simulink model "Cinematica_MGI"  (Simulink 7.7)
settings: Solver=ode45  StartTime=0.0  StopTime=inf  RelTol=1e-3
libraries: simulink x4
settings Model: Creator=JohnConstantine  LastModifiedBy=JohnConstantine

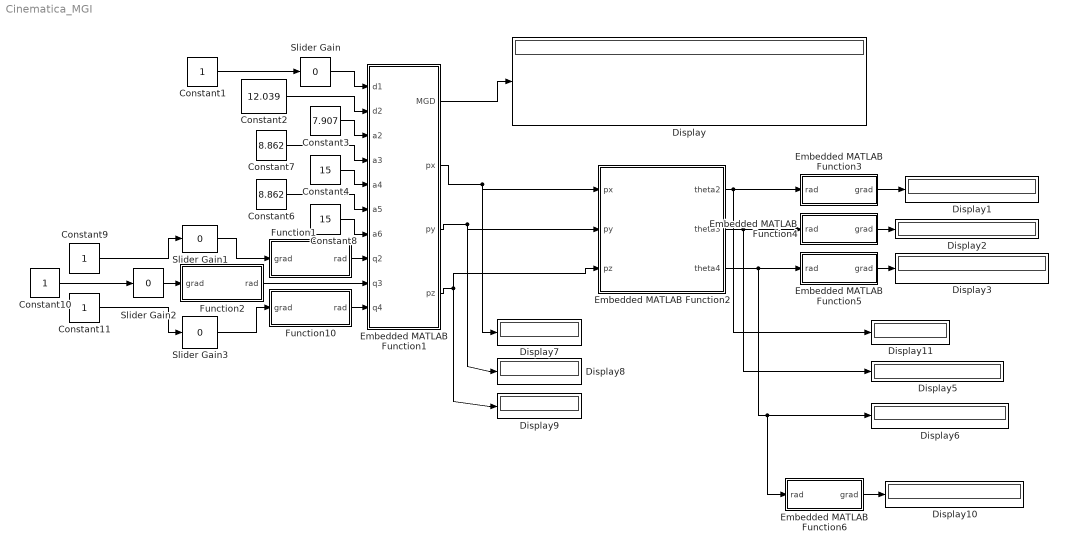
== system Cinematica_MGI ==
  Constant{1,9..11} (4 alike) : Constant
  Constant2 : Constant  Value=12.039
  Constant3 : Constant  Value=7.907
  Constant4 : Constant  Value=15
  Constant6 : Constant  Value=8.862
  Constant7 : Constant  Value=8.862
  Constant8 : Constant  Value=15
  Display{,1..3,5..11} (11 alike) : Display
  Embedded MATLAB Function1 : Stateflow chart  TreatAsAtomicUnit=on
  Embedded MATLAB Function2 : Stateflow chart  TreatAsAtomicUnit=on
  Embedded MATLAB Function3 : Stateflow chart  TreatAsAtomicUnit=on
  Embedded MATLAB Function4 : Stateflow chart  TreatAsAtomicUnit=on
  Embedded MATLAB Function5 : Stateflow chart  TreatAsAtomicUnit=on
  Embedded MATLAB Function6 : Stateflow chart  TreatAsAtomicUnit=on
  Function1 : Stateflow chart  TreatAsAtomicUnit=on
  Function10 : Stateflow chart  TreatAsAtomicUnit=on
  Function2 : Stateflow chart  TreatAsAtomicUnit=on
  Slider Gain : simulink/Math Operations/Slider Gain  SystemSampleTime=-1  low=0  gain=0  high=25
  Slider Gain1 : simulink/Math Operations/Slider Gain  SystemSampleTime=-1  low=0  gain=0  high=15
  Slider Gain2 : simulink/Math Operations/Slider Gain  SystemSampleTime=-1  low=0  gain=0  high=90
  Slider Gain3 : simulink/Math Operations/Slider Gain  SystemSampleTime=-1  low=0  gain=0  high=110
  wires:
  Embedded MATLAB Function1/2(px) -> Display7/1, Embedded MATLAB Function2/1(px)
  Embedded MATLAB Function1/1(MGD) -> Display/1
  Slider Gain/1 -> Embedded MATLAB Function1/1(d1)
  Constant4/1 -> Embedded MATLAB Function1/5(a4)
  Constant3/1 -> Embedded MATLAB Function1/3(a2)
  Constant8/1 -> Embedded MATLAB Function1/7(a6)
  Constant6/1 -> Embedded MATLAB Function1/6(a5)
  Constant7/1 -> Embedded MATLAB Function1/4(a3)
  Constant2/1 -> Embedded MATLAB Function1/2(d2)
  Embedded MATLAB Function2/1(theta2) -> Embedded MATLAB Function3/1(rad), Display11/1
  Embedded MATLAB Function2/2(theta3) -> Embedded MATLAB Function4/1(rad), Display5/1
  Embedded MATLAB Function2/3(theta4) -> Embedded MATLAB Function5/1(rad), Display6/1, Embedded MATLAB Function6/1(rad)
  Embedded MATLAB Function1/3(py) -> Display8/1, Embedded MATLAB Function2/2(py)
  Embedded MATLAB Function1/4(pz) -> Display9/1, Embedded MATLAB Function2/3(pz)
  Constant1/1 -> Slider Gain/1
  Constant9/1 -> Slider Gain1/1
  Constant10/1 -> Slider Gain2/1
  Constant11/1 -> Slider Gain3/1
  Embedded MATLAB Function3/1(grad) -> Display1/1
  Embedded MATLAB Function4/1(grad) -> Display2/1
  Embedded MATLAB Function5/1(grad) -> Display3/1
  Embedded MATLAB Function6/1(grad) -> Display10/1
  Slider Gain1/1 -> Function1/1(grad)
  Function1/1(rad) -> Embedded MATLAB Function1/8(q2)
  Function2/1(rad) -> Embedded MATLAB Function1/9(q3)
  Function10/1(rad) -> Embedded MATLAB Function1/10(q4)
  Slider Gain3/1 -> Function10/1(grad)
  Slider Gain2/1 -> Function2/1(grad)

== matlab function Embedded MATLAB Function1 ==
  data: d1 input double; MGD output double; d2 input double; a2 input double; a3 input double; a4 input double; a5 input double; a6 input double; q2 input double; q3 input double; q4 input double; px output double; py output double; pz output double
function [MGD,px,py,pz] =mgdFalange(d1,d2,a2,a3,a4,a5,a6,q2,q3,q4)

MGD= [ cos(q3)*cos(q4)*cos(pi/2 + q2) - cos(pi/2 + q2)*sin(q3)*sin(q4), - cos(q3)*cos(pi/2 + q2)*sin(q4) - cos(q4)*cos(pi/2 + q2)*sin(q3),  sin(pi/2 + q2),      a2*cos(pi/2 + q2) + cos(q3)*cos(pi/2 + q2)*(a3 + a4) + cos(q3)*cos(q4)*cos(pi/2 + q2)*(a5 + a6) - cos(pi/2 + q2)*sin(q3)*sin(q4)*(a5 + a6);...
                             - cos(q3)*sin(q4) - cos(q4)*sin(q3),                                 sin(q3)*sin(q4) - cos(q3)*cos(q4),               0,                                                                - d2 - sin(q3)*(a3 + a4) - cos(q3)*sin(q4)*(a5 + a6) - cos(q4)*sin(q3)*(a5 + a6);...
 cos(q3)*cos(q4)*sin(pi/2 + q2) - sin(q3)*sin(q4)*sin(pi/2 + q2), - cos(q3)*sin(q4)*sin(pi/2 + q2) - cos(q4)*sin(q3)*sin(pi/2 + q2), -cos(pi/2 + q2), d1 + a2*sin(pi/2 + q2) + cos(q3)*sin(pi/2 + q2)*(a3 + a4) + cos(q3)*cos(q4)*sin(pi/2 + q2)*(a5 + a6) - sin(q3)*sin(q4)*sin(pi/2 + q2)*(a5 + a6);...
                                                               0,                                                                 0,               0,                                                                                                                                               1];



% MGD=[                                                                                             cosd(theta4)*(cosd(alpha + theta2)*cosd(theta3) - sind(alpha + theta2)*cosd(alpha)*sind(theta3)) - sind(theta4)*(cosd(alpha + theta2)*sind(theta3) + sind(alpha + theta2)*cosd(alpha)*cosd(theta3)),                                                                                               - cosd(theta4)*(cosd(alpha + theta2)*sind(theta3) + sind(alpha + theta2)*cosd(alpha)*cosd(theta3)) - sind(theta4)*(cosd(alpha + theta2)*cosd(theta3) - sind(alpha + theta2)*cosd(alpha)*sind(theta3)),                                      sind(alpha + theta2)*sind(alpha),                                                                                                                                                                                 a2*cosd(alpha + theta2) + cosd(theta4)*(a5 + a6)*(cosd(alpha + theta2)*cosd(theta3) - sind(alpha + theta2)*cosd(alpha)*sind(theta3)) - sind(theta4)*(a5 + a6)*(cosd(alpha + theta2)*sind(theta3) + sind(alpha + theta2)*cosd(alpha)*cosd(theta3)) + cosd(alpha + theta2)*cosd(theta3)*(a3 + a4) - sind(alpha + theta2)*cosd(alpha)*sind(theta3)*(a3 + a4);...
%                                      cosd(theta4)*(sind(theta3)*(cosd(alpha + theta2)*cosd(alpha)^2 - sind(alpha)^2) + sind(alpha + theta2)*cosd(alpha)*cosd(theta3)) + sind(theta4)*(cosd(theta3)*(cosd(alpha + theta2)*cosd(alpha)^2 - sind(alpha)^2) - sind(alpha + theta2)*cosd(alpha)*sind(theta3)),                                     cosd(theta4)*(cosd(theta3)*(cosd(alpha + theta2)*cosd(alpha)^2 - sind(alpha)^2) - sind(alpha + theta2)*cosd(alpha)*sind(theta3)) - sind(theta4)*(sind(theta3)*(cosd(alpha + theta2)*cosd(alpha)^2 - sind(alpha)^2) + sind(alpha + theta2)*cosd(alpha)*cosd(theta3)), - cosd(alpha)*sind(alpha) - cosd(alpha + theta2)*cosd(alpha)*sind(alpha),                                                            a2*sind(alpha + theta2)*cosd(alpha) - d2*sind(alpha) + sind(theta3)*(cosd(alpha + theta2)*cosd(alpha)^2 - sind(alpha)^2)*(a3 + a4) + cosd(theta4)*(a5 + a6)*(sind(theta3)*(cosd(alpha + theta2)*cosd(alpha)^2 - sind(alpha)^2) + sind(alpha + theta2)*cosd(alpha)*cosd(theta3)) + sind(theta4)*(a5 + a6)*(cosd(theta3)*(cosd(alpha + theta2)*cosd(alpha)^2 - sind(alpha)^2) - sind(alpha + theta2)*cosd(alpha)*sind(theta3)) + sind(alpha + theta2)*cosd(alpha)*cosd(theta3)*(a3 + a4);...
%  cosd(theta4)*(sind(theta3)*(cosd(alpha)*sind(alpha) + cosd(alpha + theta2)*cosd(alpha)*sind(alpha)) + sind(alpha + theta2)*sind(alpha)*cosd(theta3)) + sind(theta4)*(cosd(theta3)*(cosd(alpha)*sind(alpha) + cosd(alpha + theta2)*cosd(alpha)*sind(alpha)) - sind(alpha + theta2)*sind(alpha)*sind(theta3)), cosd(theta4)*(cosd(theta3)*(cosd(alpha)*sind(alpha) + cosd(alpha + theta2)*cosd(alpha)*sind(alpha)) - sind(alpha + theta2)*sind(alpha)*sind(theta3)) - sind(theta4)*(sind(theta3)*(cosd(alpha)*sind(alpha) + cosd(alpha + theta2)*cosd(alpha)*sind(alpha)) + sind(alpha + theta2)*sind(alpha)*cosd(theta3)),                     cosd(alpha)^2 - cosd(alpha + theta2)*sind(alpha)^2, d1 + d2*cosd(alpha) + a2*sind(alpha + theta2)*sind(alpha) + sind(theta3)*(a3 + a4)*(cosd(alpha)*sind(alpha) + cosd(alpha + theta2)*cosd(alpha)*sind(alpha)) + cosd(theta4)*(a5 + a6)*(sind(theta3)*(cosd(alpha)*sind(alpha) + cosd(alpha + theta2)*cosd(alpha)*sind(alpha)) + sind(alpha + theta2)*sind(alpha)*cosd(theta3)) + sind(theta4)*(a5 + a6)*(cosd(theta3)*(cosd(alpha)*sind(alpha) + cosd(alpha + theta2)*cosd(alpha)*sind(alpha)) - sind(alpha + theta2)*sind(alpha)*sind(theta3)) + sind(alpha + theta2)*sind(alpha)*cosd(theta3)*(a3 + a4);...
%                                                                                                                                                                                                                                                                                        0,                                                                                                                                                                                                                                                                                       0,                                                                   0,                                                                                                                                                                                                                                                                                                                                                                                                                                                                                                                       1];
% 
% 
            px=MGD(1,4);
            py=MGD(2,4);
            pz=MGD(3,4);

== matlab function Embedded MATLAB Function2 ==
  data: px input double; py input double; pz input double; theta2 output double; theta3 output double; theta4 output double
function [theta2,theta3,theta4] =mgIFalange(px,py,pz)


a2=7.907;
a3=8.862;
a4=15;
a5=8.862;
a6=15;
a34=a3+a4;
a56=a5+a6;

r= sqrt(px^2+pz^2);
r_a2= r-a2;

%
theta2=atan(px/pz);
% 
    ctheta4n=(px^2+py^2+pz^2-a34^2-a56^2);
    cthetad=2*a34*a56;
    Ctheta4=(ctheta4n/cthetad)%
   % theta4=acos(complex((px^2+pz^2+py^2-a34^2-a56^2)/2*a34*a56))
    Stheta4=sqrt(complex(1-(Ctheta4)^2))
%
theta4=atan(Stheta4/Ctheta4)
%
    B=atan(py/r_a2)
    alpha=atan((a56*Stheta4)/((a34+a56)*Ctheta4)) 
%   
 theta3=B-alpha
%


% r= sqrt(Px^2+Pz^2);
% r_a2=r-a2;
% l=sqrt(r_a2^2+Py^2);
% 
% phi=atan(Py/r_a2);
% B=acos((l^2+a34^2-a56^2)/(2*l*a34));
% b=abs(B);
% psi=acos((a34^2+a56^2-l^2)/(2*a34*a56));
% psis=abs(psi);
% 
% theta2=atan(Px/Pz);
% theta3=phi-B;
% theta4=pi-psi;
%

== matlab function Embedded MATLAB Function4 ==
  data: rad input double; grad output double
function grad=rad_to_grad(rad)

grad=(rad*180)/pi;

== matlab function Embedded MATLAB Function5 ==
  data: rad input double; grad output double
function grad=rad_to_grad(rad)

grad= ((rad*180)/pi);

== matlab function Embedded MATLAB Function3 ==
  data: rad input double; grad output double
function grad=rad_to_grad(rad)

grad=(rad*180)/pi;

== matlab function Function1 ==
  data: grad input double; rad output double
function rad =grad2rad(grad)

rad=grad*2*pi/360;

== matlab function Function2 ==
  data: grad input double; rad output double
function rad =grad2rad(grad)

rad=grad*2*pi/360;

== matlab function Embedded MATLAB Function6 ==
  data: rad input double; grad output double
function grad=rad_to_grad(rad)

grad= abs(rad);

== matlab function Function10 ==
  data: grad input double; rad output double
function rad =grad2rad(grad)

rad=grad*2*pi/360;
